simulink model "simulink4"  (R2015a)
settings: Solver=ode45  StartTime=0.0  StopTime=20.0  RelTol=1e-3
values from neighbouring files (symbols this model uses):
  sys = (10*s + 1)/((s + 1)*(2*s+1))    [lez4.m]
  systd = c2d(sys, Ts, 'zoh')    [lez4.m]
  Ts = 1/10    (= 0.1)    [lez4.m]
settings Model: Creator=lezione00  LastModifiedBy=lezione00

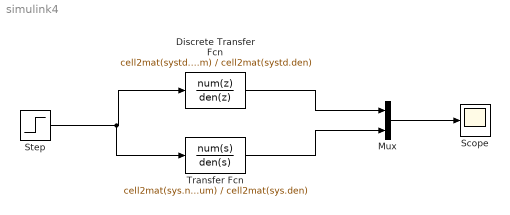
== system simulink4 ==
  Discrete Transfer Fcn : DiscreteTransferFcn  Numerator=cell2mat(systd.num)  Denominator=cell2mat(systd.den)  SampleTime=Ts
  Mux : Mux  Inputs=2
  Scope : Scope
  Step : Step  SampleTime=0
  Transfer Fcn : TransferFcn  Numerator=cell2mat(sys.num)  Denominator=cell2mat(sys.den)
  wires:
  Mux/1 -> Scope/1
  Step/1 -> Transfer Fcn/1, Discrete Transfer Fcn/1
  Discrete Transfer Fcn/1 -> Mux/1
  Transfer Fcn/1 -> Mux/2
